simulink model "esp32_adc_demo"  (R2022a)
settings: Solver=FixedStepDiscrete  StartTime=0.0  StopTime=10.0  RelTol=1e-3  EnableMultiTasking=on
undefined symbols (not defined in the file): ESP, IDF
libraries: esp32_io_lib x3, simulink x1, esp32_device_config_lib x1
settings Model: Creator=dhanika  LastModifiedBy=62-603
settings SolverCC: AlgebraicLoopSolver=TrustRegion  PositivePriorityOrder=on  AutoInsertRateTranBlk=on
settings DataIOCC: ReturnWorkspaceOutputs=off
settings OptimizationCC: DefaultParameterBehavior=Inlined  EnhancedBackFolding=on  PassReuseOutputArgsAs=Individual arguments  OptimizeBlockOrder=speed  DifferentSizesBufferReuse=on  OptimizationCustomize=off  EfficientTunableParamExpr=on
settings DebuggingCC: ParameterTunabilityLossMsg=error  UnconnectedInputMsg=warning  UnconnectedOutputMsg=warning  UnconnectedLineMsg=warning  SFMachineParentedDataDiag=warning  ArithmeticOperatorsInVariantConditions=warning
settings HardwareCC: ProdBitPerPointer=32  ProdBitPerSizeT=32  ProdBitPerPtrDiffT=32  ProdLargestAtomicFloat=None  ProdIntDivRoundTo=Undefined  ProdEndianess=Unspecified  ProdWordSize=32  ProdHWDeviceType=Cadence Design Systems (Tensilica)->Xtensa® single-/dual-core 32-bit LX6 microprocessor
settings SFSimCC: MATLABDynamicMemAlloc=off  CustomCodeUndefinedFunction=UseInterfaceOnly
settings RTWCC: Description=Waijung 2 ESP32 target  SystemTargetFile=esp32.tlc  GenCodeOnly=on  MakeCommand=make_rtw TMF=1  GenerateMakefile=off  TemplateMakefile=ert_default_tmf  GenerateReport=on  RetainRTWFile=on  IncludeHyperlinkInReport=on  LaunchReport=on  GenerateTraceInfo=on  GenerateTraceReport=on  GenerateTraceReportSl=on  GenerateTraceReportSf=on  GenerateTraceReportEml=on
settings CodeAppCC: ForceParamTrailComments=on  IgnoreCustomStorageClasses=off  OperatorAnnotations=on  SimulinkDataObjDesc=on  SFDataObjDesc=on  InsertBlockDesc=on
settings ERTTargetCC: TargetLangStandard=C99 (ISO)  UseToolchainInfoCompliant=off  InlinedParameterPlacement=NonHierarchical  ERTSrcFileBannerTemplate=esp32_code_template.cgt  ERTHdrFileBannerTemplate=esp32_code_template.cgt  ERTDataSrcFileTemplate=esp32_code_template.cgt  ERTDataHdrFileTemplate=esp32_code_template.cgt  ERTCustomFileTemplate=esp32_file_process.tlc

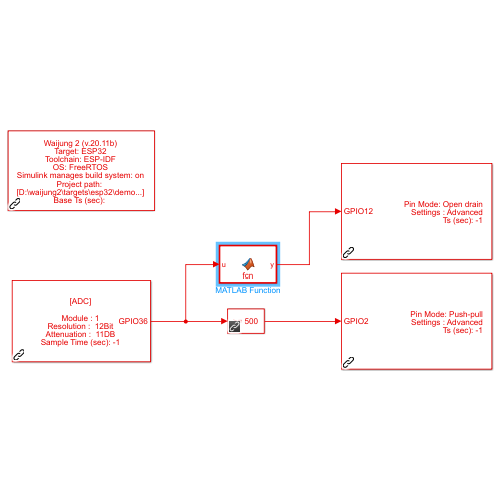
[thumbnail: Simulink's stored preview of the top-level diagram]
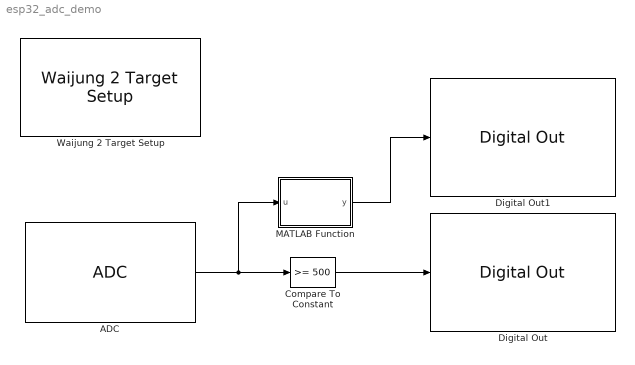
== system esp32_adc_demo ==
  ADC : esp32_io_lib/ADC  blockid=ADC  adcmodule=1  adcresolution=12Bit  adcatten=11DB  outputdatatype=Double  pin32=off  pin33=off  pin34=off  pin35=off  pin36=on  pin37=off  pin38=off  pin39=off  pin0=off  pin2=on  pin4=on  pin12=on  pin13=off  pin14=off  pin15=off  pin25=off  pin26=off  pin27=off  sampletime=-1  pinarray1="[0  0  0  0  1  0  0  0]"  pinarray2="[0  1  1  1  0  0  0  0  0  0]"  adcresolutiondef=ADC_WIDTH_BIT_12  adcattendef=ADC_ATTEN_DB_11  pinoutcount1=1  pinoutcount2=3  pinstring1="[\"ADC1_CHANNEL_4\",\"ADC1_CHANNEL_5\",\"ADC1_CHANNEL_6\",\"ADC1_CHANNEL_7\",\"ADC1_CHANNEL_0\",\"ADC1_CHANNEL_1\",\"ADC1_CHANNEL_2\",\"ADC1_CHANNEL_3\"]"  pinstring2="[\"ADC2_CHANNEL_1\",\"ADC2_CHANNEL_2\",\"ADC2_CHANNEL_0\",\"ADC2_CHANNEL_5\",\"ADC2_CHANNEL_4\",\"ADC2_CHANNEL_6\",\"ADC2_CHANNEL_3\",\"ADC2_CHANNEL_8\",\"ADC2_CHANNEL_9\",\"ADC2_CHANNEL_7\"]"  pinname1="[\"GPIO32\",\"GPIO33\",\"GPIO34\",\"GPIO35\",\"GPIO36\",\"GPIO37\",\"GPIO38\",\"GPIO39\"]"  pinname2="[\"GPIO0\",\"GPIO2\",\"GPIO4\",\"GPIO12\",\"GPIO13\",\"GPIO14\",\"GPIO15\",\"GPIO25\",\"GPIO26\",\"GPIO27\"]"
      settings: SourceProductName=Waijung 2 Blockset
  Compare To Constant : simulink/Logic and Bit Operations/Compare To Constant  relop=>=  const=500  OutDataTypeStr=boolean
  Digital Out : esp32_io_lib/Digital Out  blockid=DigitalOut  settings=Advanced  pin0=off  pin1=off  pin2=on  pin3=off  pin4=off  pin5=off  pin6=off  pin7=off  pin8=off  pin9=off  pin10=off  pin11=off  pin12=off  pin13=off  pin14=off  pin15=off  pin16=off  pin17=off  pin18=off  pin19=off  pin20=off  pin21=off  pin22=off  pin23=off  pin24=off  pin25=off  pin26=off  pin27=off  pin28=off  pin29=off  pin30=off  pin31=off  pin32=off  pin33=off  pin34=off  pin35=off  pin36=off  pin37=off  pin38=off  pin39=off  pin40=off  pin41=off  pin42=off  pin43=off  pin44=off  pin45=off  pin_initialize=on  pin_mode=Push-pull  sampletime=-1  drive_capability=Normal (default)  pin_hold=Disable  deep_sleep_pin_hold=Disable  pin_array="[0  0  1  0  0  0  0  0  0  0  0  0  0  0  0  0  0  0  0  0  0  0  0  0  0  0  0  0  0  0  0  0  0  0  0  0  0  0  0  0  0  0  0  0  0  0]"  inport_num=1  drive_capability_define=GPIO_DRIVE_CAP_2  pin_hold_define=off  pin_mode_define=GPIO_MODE_OUTPUT  deep_sleep_pin_hold_define=off  pin_string=((1ULL<<2))
      settings: SourceProductName=Waijung 2 Blockset
  Digital Out1 : esp32_io_lib/Digital Out  blockid=DigitalOut1  settings=Advanced  pin0=off  pin1=off  pin2=off  pin3=off  pin4=off  pin5=off  pin6=off  pin7=off  pin8=off  pin9=off  pin10=off  pin11=off  pin12=on  pin13=off  pin14=off  pin15=off  pin16=off  pin17=off  pin18=off  pin19=off  pin20=off  pin21=off  pin22=off  pin23=off  pin24=off  pin25=off  pin26=off  pin27=off  pin28=off  pin29=off  pin30=off  pin31=off  pin32=off  pin33=off  pin34=off  pin35=off  pin36=off  pin37=off  pin38=off  pin39=off  pin40=off  pin41=off  pin42=off  pin43=off  pin44=off  pin45=off  pin_initialize=on  pin_mode=Open drain  sampletime=-1  drive_capability=Normal (default)  pin_hold=Disable  deep_sleep_pin_hold=Disable  pin_array="[0  0  0  0  0  0  0  0  0  0  0  0  1  0  0  0  0  0  0  0  0  0  0  0  0  0  0  0  0  0  0  0  0  0  0  0  0  0  0  0  0  0  0  0  0  0]"  inport_num=1  drive_capability_define=GPIO_DRIVE_CAP_2  pin_hold_define=off  pin_mode_define=GPIO_MODE_OUTPUT_OD  deep_sleep_pin_hold_define=off  pin_string=((1ULL<<12))
      settings: SourceProductName=Waijung 2 Blockset
  MATLAB Function : MATLAB Function  TreatAsAtomicUnit=on
  Waijung 2 Target Setup : esp32_device_config_lib/Waijung 2 Target Setup  toolchain=ESP-IDF  os=FreeRTOS  sampletime=-1  simulink_managebuildsystem=on  projectpath=D:\waijung2\targets\esp32\demo\adc_demo\esp32_adc_demo_esp32_build_system  espidfpath=C:\msys32\home\skris\esp\esp-idf  auto_compile_download=on  blockid=Waijung2TargetSetup  target=ESP32  waijungversion=20.11b  defaultstacksize=2048  basepriority=0  highestpriority=16  generate_baserate_task=on  esp32flashsize=4MB  esp32comport=COM3
      settings: SourceProductName=Waijung 2 Blockset
  wires:
  ADC/1 -> MATLAB Function/1(u), Compare To Constant/1
  Compare To Constant/1 -> Digital Out/1
  MATLAB Function/1(y) -> Digital Out1/1

== matlab function esp32_adc_demo/MATLAB Function ==
  data: u input; y output
function y = fcn(u)

if u >= 500
    y = true;
else
    y = false;
end
